simulink model "Model_RB_APF_WF_VO_original"  (R2024b)
settings: Solver=FixedStepAuto  StartTime=0.0  StopTime=120  FixedStep=UAVSampleTime  RelTol=1e-3
undefined symbols (not defined in the file): DroneMass, Gravity, Horizontal_Limits, Horizontal_Res, kD_pos, kD_vel, kI_pos, kI_vel, kP_pos, kP_vel, Lidar, MaxRange, N_filter, TopSpeed, UAV, Vertical_Limits, Vertical_Res, Waypoints
libraries: slpidlib x6, uavsimlib x4, robotcorelib x1, uavalgslib x1
(part 2 of 2)

== matlab function Model_RB_APF_WF_VO_original/Path Planning Data/VOActivator_V5 ==
  settings: updateMethod=DISCRETE
  data: Minima_list input; Minima_count input; position input; Virtuals_list output; flight_mode input; Virtuals_count output; t input
function [Virtuals_list, Virtuals_count] = VOActivator(Minima_list, Minima_count, position, flight_mode, t)

activation_dist = 3;
maxVO = 100;

persistent VO_list
persistent VO_count
persistent next_to_check
persistent was_in_WF

if isempty(VO_list)
    VO_list      = zeros(maxVO, 3);
    VO_count     = 0;
    next_to_check = 1;
    was_in_WF     = false(maxVO, 1);

    % Pass to workspace at least once
    assignin('base', 'finalVOList',  VO_list);
    assignin('base', 'finalVOCount', VO_count);
    
end

% Mark all current unactivated minima as having been in WF
if flight_mode == 2 || flight_mode == 3
    was_in_WF(next_to_check:Minima_count) = true;
end

% Check unactivated minima for activation
for i = next_to_check:Minima_count
    d = norm(position(:) - Minima_list(i,:).');
    if d > activation_dist || (flight_mode == 1 && was_in_WF(i))
        % VO is activated
        %disp("VO Activated at t ="); disp(t);
        VO_count = VO_count + 1;
        VO_list(VO_count, :) = Minima_list(i,:);
        next_to_check = i + 1;
        % Update VO list in workspace
        assignin('base', 'finalVOList',  VO_list);
        assignin('base', 'finalVOCount', VO_count);
    end
end

Virtuals_list  = VO_list;
Virtuals_count = VO_count;

== matlab function Model_RB_APF_WF_VO_original/Path Planning Data/GoalReached_V5 ==
  settings: updateMethod=DISCRETE
  data: time input; currentWaypoint output; endSim output; pos input; waypoints input
function [currentWaypoint, endSim] = fcn(time, pos, waypoints)

waypoint_threshold = 0.25;

persistent idx;
persistent numWaypoints;
if isempty(idx)
    idx = 1;
    numWaypoints = size(waypoints, 1);
end

if norm(waypoints(idx,:).' - pos) < waypoint_threshold
    disp('Reached Waypoint');
    disp(idx);
    idx = idx + 1;
end

if idx > numWaypoints
    endSim = 1;
    currentWaypoint = waypoints(end,:).'; % can't have it empty
    disp('Sim ended at t =');
    disp(time);
    return;
end

currentWaypoint = waypoints(idx,:).';
endSim = 0;

== matlab function Model_RB_APF_WF_VO_original/Controller/MATLAB Function1 ==
  data: vel_cmd input; vel_capped output; TopSpeed input
function vel_capped = limiter(vel_cmd, TopSpeed)

mag = norm(vel_cmd);

if mag > TopSpeed
    vel_capped = TopSpeed*(vel_cmd/mag);
else
    vel_capped = vel_cmd;
end

== matlab function Model_RB_APF_WF_VO_original/WF/MATLAB Function1 ==
  data: WF_vec input; WF_VecCapped output
function WF_VecCapped = limiter(WF_vec)

maximum = 5;

mag = norm(WF_vec);

if mag > maximum
    WF_VecCapped = maximum*(WF_vec/mag);
else
    WF_VecCapped = WF_vec;
end

== matlab function Model_RB_APF_WF_VO_original/WF/WFVectors ==
  data: cloud input; virtuals input; virtualCount input; flight_mode input; radial_vec output; lateral_vec output; pos input
function [radial_vec, lateral_vec] = WF(cloud, virtuals, virtualCount, flight_mode, pos)

% Parameters
comfort_zone = 2;
lateral_scaler = 0.5;
radial_scaler = 0.8;

% Initializations
n_points = size(cloud,1);
d_min = inf;                    % initialize with very large number
r_min = zeros(3,1);             % closest-point vector (radial)

% Loop through lidar points for closest point
for i = 1:n_points
    % Per particular pixel/ray

    r = -cloud(i,:).';         % 3x1 vector of distance 
    D = norm(r);               % scalar distance

    % check if this is the closest so far
    if D < d_min
        d_min = D;
        r_min = r;
    end
end

% Loop through VOs for closest point
for i = 1:virtualCount
    r = -(virtuals(i,1:3).' - pos);
    D = norm(r);
    % check if this is the closest so far
    if D < d_min
        d_min = D;
        r_min = r;
    end
end

% Radial
radial_dir = r_min / d_min;             % unit vector
radial_dif = (comfort_zone - d_min);
radial_vec = radial_dir*radial_dif*radial_scaler;

% Lateral
if flight_mode == 2
    rotation = -pi/2;   % Go Left
else
    rotation = pi/2;    % Go right
end

lateral_dir = axang2rotm([0 0 1 rotation])*radial_dir;  % this is rotating about z axis, not exactly orthogonal to raidal_vec
lateral_vec = lateral_dir*lateral_scaler;
